simulink model "control_filtro_dq_mod2"  (R2017b)
settings: Solver=ode1  StartTime=0.0  StopTime=0.5  FixedStep=Ts  MaxStep=1e-4  RelTol=1e-3
InitFcn:
  | GlobalParam
values from neighbouring files (symbols this model uses):
  APFon = 0.025    [GlobalParam.m]
  Cdc = 680e-6    (= 0.00068)    [GlobalParam.m]
  fc = 15000    [GlobalParam.m]
  fe = 50    [GlobalParam.m]
  Ideal = 0    [GlobalParam.m]
  Lf = 0.01    [GlobalParam.m]
  LL = 0.055462    [GlobalParam.m]
  nc = 3    [GlobalParam.m]
  Rf = 0.35    [GlobalParam.m]
  RL = 23.232    [GlobalParam.m]
  teta_a = 0    [GlobalParam.m]
  teta_b = 120    [GlobalParam.m]
  teta_c = -120    [GlobalParam.m]
  Tm = 1/fm    (= 5e-05)    [GlobalParam.m]
  Ts = 5e-6    (= 5e-06)    [GlobalParam.m]
  Vdc = 62    [GlobalParam.m]
  Vs = 120*sqrt(2)    [GlobalParam.m]
libraries: powerlib x106, simulink x10, cstblocks x3, peTransforms x2, peSinusoidalMeasurement x1, powerlib_meascontrol x1
(part 1 of 2)
settings Model: Creator=user  LastModifiedBy=user

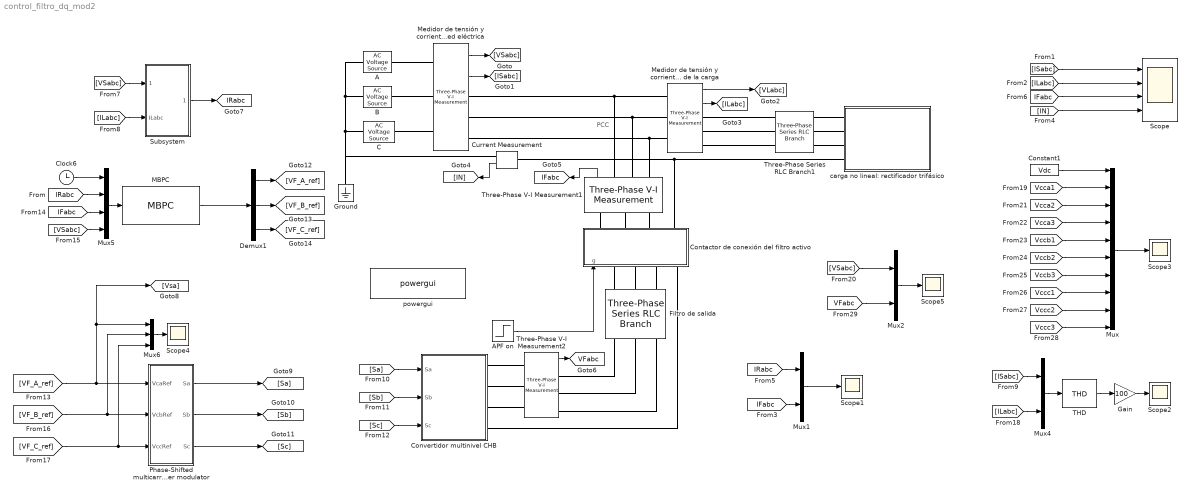
== system control_filtro_dq_mod2 ==
  note: PCC
  "A " : powerlib/Electrical Sources/AC Voltage Source  Amplitude=Vs  Phase=teta_a  Frequency=fe  SampleTime=0  Measurements=None  BusType=swing  Pref=10e3  Qref=0  Qmin=-inf  Qmax=+inf
  APF on : Step  Time=APFon  SampleTime=0
  "B " : powerlib/Electrical Sources/AC Voltage Source  Amplitude=Vs  Phase=teta_b  Frequency=fe  SampleTime=0  Measurements=None  BusType=swing  Pref=10e3  Qref=0  Qmin=-inf  Qmax=+inf
  "C " : powerlib/Electrical Sources/AC Voltage Source  Amplitude=Vs  Phase=teta_c  Frequency=fe  SampleTime=0  Measurements=None  BusType=swing  Pref=10e3  Qref=0  Qmin=-inf  Qmax=+inf
  Clock6 : Clock
  Constant1 : Constant  Value=Vdc
  "Contactor de conexión del filtro activo " : Subsystem
  Convertidor multinivel CHB : Subsystem
  Current Measurement : powerlib/Measurements/Current Measurement  PhasorSimulation=off  OutputType=Complex  PSBequivalent=0
  Demux1 : Demux  Outputs=3
  Filtro de salida : powerlib/Elements/Three-Phase Series RLC Branch  LConnTagsString=A|B|C  RConnTagsString=A|B|C  BranchType=RL  Resistance=Rf  Inductance=Lf  Capacitance=1e-6  Measurements=None
  Gain : Gain  Gain=100
  Ground : powerlib/Elements/Ground  LConnTagsString=a
  MBPC : MATLABFcn  MATLABFcn=MBPC  OutputDimensions=3
  Medidor de tensión y corriente de la red eléctrica : powerlib/Measurements/Three-Phase V-I Measurement  VoltageMeasurement=phase-to-ground  SetLabelV=off  LabelV=Vabc  Vpu=off  VpuLL=off  CurrentMeasurement=yes  SetLabelI=off  LabelI=Iabc  Ipu=off  Pbase=100e6  Vbase=500e3  OutputType=Complex  PhasorSimulation=off  PSBequivalent=0
  "Medidor de tensión y corriente de la carga " : powerlib/Measurements/Three-Phase V-I Measurement  VoltageMeasurement=phase-to-ground  SetLabelV=off  LabelV=Vabc  Vpu=off  VpuLL=off  CurrentMeasurement=yes  SetLabelI=off  LabelI=Iabc  Ipu=off  Pbase=100e6  Vbase=500e3  OutputType=Complex  PhasorSimulation=off  PSBequivalent=0
  Mux : Mux  Inputs=10
  Mux1 : Mux  Inputs=2
  Mux2 : Mux  Inputs=2
  Mux4 : Mux  Inputs=2
  Mux5 : Mux
  Mux6 : Mux  Inputs=3
  Phase-Shifted multicarrier modulator : Subsystem
  Scope : Scope  NumInputPorts=4
  Scope{1..5} (5 alike) : Scope
  Subsystem : Subsystem
  THD : powerlib_meascontrol/Measurements/THD  Freq=50  Ts=Ts
  Three-Phase Series RLC Branch1 : powerlib/Elements/Three-Phase Series RLC Branch  LConnTagsString=A|B|C  RConnTagsString=A|B|C  BranchType=RL  Resistance=0.09  Inductance=0.001  Capacitance=1e-6  Measurements=None
  Three-Phase V-I Measurement1 : powerlib/Measurements/Three-Phase V-I Measurement  VoltageMeasurement=no  SetLabelV=off  LabelV=Vabc  Vpu=off  VpuLL=off  CurrentMeasurement=yes  SetLabelI=off  LabelI=Iabc  Ipu=off  Pbase=100e6  Vbase=500e3  OutputType=Complex  PhasorSimulation=off  PSBequivalent=0
  Three-Phase V-I Measurement2 : powerlib/Measurements/Three-Phase V-I Measurement  VoltageMeasurement=phase-to-ground  SetLabelV=off  LabelV=Vabc  Vpu=off  VpuLL=off  CurrentMeasurement=no  SetLabelI=off  LabelI=Iabc  Ipu=off  Pbase=100e6  Vbase=500e3  OutputType=Complex  PhasorSimulation=off  PSBequivalent=0
  "carga no lineal: rectificador trifásico " : Subsystem
  powergui : powerlib/powergui  Priority=1  SimulationMode=Discrete  SampleTime=Ts  frequency=60  Iterations=50  frequencyindice=50  Pbase=100e6  ErrMax=1e-4  UnitsV=kV  UnitsW=MW  buscounter=0  FunctionMessages=off  echomessages=off  EnableUseOfTLC=off  CurrentSourceSwitches=off  DisableSnubberDevices=off  DisableRonSwitches=off  DisableVfSwitches=off  DisplayEquations=off  SolverType=Tustin/Backward Euler (TBE)  Interpol=off  ExternalGateDelay=off  methode=off  Ts=100  x0status=blocks  SPID=on  SwTol=0  HookPort=off  RestoreLinks=warning  ResistiveCurrentMeasurement=off  Frange=[0:2:500]  Ylog=off  Xlog=on  ShowGrid=off  save=off  variable=ZData  structure=vg11  ZoomFFT=off  StartTime=0.04  cycles=2  DisplayStyle=1  fundamental=50  FreqAxis=on  MaxFrequency=30000  frequencyindicesteady=1  RmsSteady=1  display=off
  tag scope: IFabc=global, IRabc=global, VFabc=global
  wires:
  Medidor de tensión y corriente de la red eléctrica/1 -> [VSabc]
  Medidor de tensión y corriente de la red eléctrica/2 -> [ISabc]
  "Medidor de tensión y corriente de la carga "/1 -> [VLabc]
  "Medidor de tensión y corriente de la carga "/2 -> [ILabc]
  [ILabc] -> Scope/2
  APF on/1 -> "Contactor de conexión del filtro activo "/1(g)
  Current Measurement/1 -> [IN]
  Three-Phase V-I Measurement1/1 -> [IFabc]
  Three-Phase V-I Measurement2/1 -> [VFabc]
  Mux5/1 -> MBPC/1
  MBPC/1 -> Demux1/1
  Clock6/1 -> Mux5/1
  [IRabc] -> Mux5/2
  [VSabc] -> Mux5/4
  [Sa] -> Convertidor multinivel CHB/1(Sa)
  [Sb] -> Convertidor multinivel CHB/2(Sb)
  [Sc] -> Convertidor multinivel CHB/3(Sc)
  [IFabc] -> Scope/3
  [IN] -> Scope/4
  [ISabc] -> Scope/1
  [IFabc] -> Mux5/3
  [IFabc] -> Mux1/2
  [IRabc] -> Mux1/1
  Mux1/1 -> Scope1/1
  [ISabc] -> Mux4/1
  Mux4/1 -> THD/1
  [ILabc] -> Mux4/2
  [Vccc1] -> Mux/8
  [Vcca1] -> Mux/2
  Constant1/1 -> Mux/1
  [Vccc2] -> Mux/9
  [Vccb2] -> Mux/6
  [Vccb1] -> Mux/5
  [Vccc3] -> Mux/10
  Mux/1 -> Scope3/1
  [Vccb3] -> Mux/7
  [Vcca3] -> Mux/4
  [Vcca2] -> Mux/3
  Demux1/1 -> [VF_A_ref]
  Demux1/2 -> [VF_B_ref]
  Demux1/3 -> [VF_C_ref]
  [VSabc] -> Mux2/1
  Mux2/1 -> Scope5/1
  THD/1 -> Gain/1
  Gain/1 -> Scope2/1
  [ILabc] -> Subsystem/2("ILabc ")
  [VSabc] -> Subsystem/1("VSabc ")
  Subsystem/1(IRabc1) -> [IRabc]
  [VFabc] -> Mux2/2
  Phase-Shifted multicarrier modulator/3(Sc) -> [Sc]
  Phase-Shifted multicarrier modulator/1(Sa) -> [Sa]
  Phase-Shifted multicarrier modulator/2(Sb) -> [Sb]
  Mux6/1 -> Scope4/1
  [VF_C_ref] -> Mux6/3, Phase-Shifted multicarrier modulator/3(VccRef)
  [VF_B_ref] -> Mux6/2, Phase-Shifted multicarrier modulator/2(VcbRef)
  [VF_A_ref] -> [Vsa], Mux6/1, Phase-Shifted multicarrier modulator/1(VcaRef)
  connections:
  "C "/LConn1 -- Ground/LConn1 -- Current Measurement/RConn1 -- "A "/LConn1 -- "B "/LConn1
  Medidor de tensión y corriente de la red eléctrica/LConn2 -- "B "/RConn1
  Medidor de tensión y corriente de la red eléctrica/LConn3 -- "C "/RConn1
  Medidor de tensión y corriente de la red eléctrica/LConn1 -- "A "/RConn1
  "Medidor de tensión y corriente de la carga "/LConn1 -- Three-Phase V-I Measurement1/RConn1 -- Medidor de tensión y corriente de la red eléctrica/RConn1
  "Medidor de tensión y corriente de la carga "/LConn2 -- Three-Phase V-I Measurement1/RConn2 -- Medidor de tensión y corriente de la red eléctrica/RConn2
  Medidor de tensión y corriente de la red eléctrica/RConn3 -- "Medidor de tensión y corriente de la carga "/LConn3 -- Three-Phase V-I Measurement1/RConn3
  Three-Phase Series RLC Branch1/LConn1 -- "Medidor de tensión y corriente de la carga "/RConn1
  Three-Phase Series RLC Branch1/LConn2 -- "Medidor de tensión y corriente de la carga "/RConn2
  Three-Phase Series RLC Branch1/LConn3 -- "Medidor de tensión y corriente de la carga "/RConn3
  Filtro de salida/RConn1 -- "Contactor de conexión del filtro activo "/LConn1
  "Contactor de conexión del filtro activo "/LConn2 -- Filtro de salida/RConn2
  Filtro de salida/RConn3 -- "Contactor de conexión del filtro activo "/LConn3
  Current Measurement/LConn1 -- "carga no lineal: rectificador trifásico "/LConn4 -- "Contactor de conexión del filtro activo "/RConn4
  Three-Phase V-I Measurement2/RConn1 -- Filtro de salida/LConn1
  Three-Phase V-I Measurement2/RConn2 -- Filtro de salida/LConn2
  Three-Phase V-I Measurement2/RConn3 -- Filtro de salida/LConn3
  Three-Phase V-I Measurement2/LConn1 -- Convertidor multinivel CHB/RConn1
  Three-Phase V-I Measurement2/LConn2 -- Convertidor multinivel CHB/RConn2
  Three-Phase V-I Measurement2/LConn3 -- Convertidor multinivel CHB/RConn3
  "Contactor de conexión del filtro activo "/LConn4 -- Convertidor multinivel CHB/RConn4
  "Contactor de conexión del filtro activo "/RConn3 -- Three-Phase V-I Measurement1/LConn3
  "Contactor de conexión del filtro activo "/RConn2 -- Three-Phase V-I Measurement1/LConn2
  "Contactor de conexión del filtro activo "/RConn1 -- Three-Phase V-I Measurement1/LConn1
  "carga no lineal: rectificador trifásico "/LConn1 -- Three-Phase Series RLC Branch1/RConn1
  "carga no lineal: rectificador trifásico "/LConn2 -- Three-Phase Series RLC Branch1/RConn2
  Three-Phase Series RLC Branch1/RConn3 -- "carga no lineal: rectificador trifásico "/LConn3

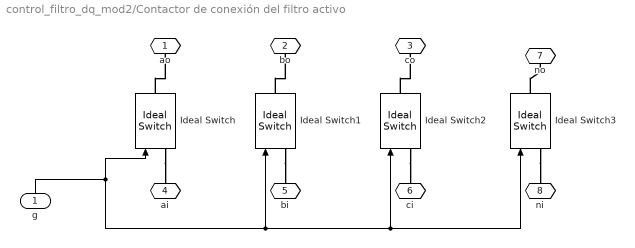
== system control_filtro_dq_mod2/Contactor de conexión del filtro activo  ==
  g : Inport
  Ideal Switch{,1..3} (4 alike) : powerlib/Power Electronics/Ideal Switch  Ron=0.001  Lon=0  IC=0  Rs=1e5  Cs=inf  Measurements=off
  ao : PMIOPort  Port=1  Side=Right
  bo : PMIOPort  Port=2  Side=Right
  co : PMIOPort  Port=3  Side=Right
  ai : PMIOPort  Port=4  Side=Left
  bi : PMIOPort  Port=5  Side=Left
  ci : PMIOPort  Port=6  Side=Left
  no : PMIOPort  Port=7  Side=Left
  ni : PMIOPort  Port=8  Side=Right
  wires:
  g/1 -> Ideal Switch3/1, Ideal Switch2/1, Ideal Switch1/1, Ideal Switch/1
  connections:
  Ideal Switch1/RConn1 -- bo/RConn1
  Ideal Switch1/LConn1 -- bi/RConn1
  Ideal Switch/RConn1 -- ao/RConn1
  Ideal Switch2/RConn1 -- co/RConn1
  Ideal Switch2/LConn1 -- ci/RConn1
  Ideal Switch/LConn1 -- ai/RConn1
  Ideal Switch3/LConn1 -- ni/RConn1
  Ideal Switch3/RConn1 -- no/RConn1

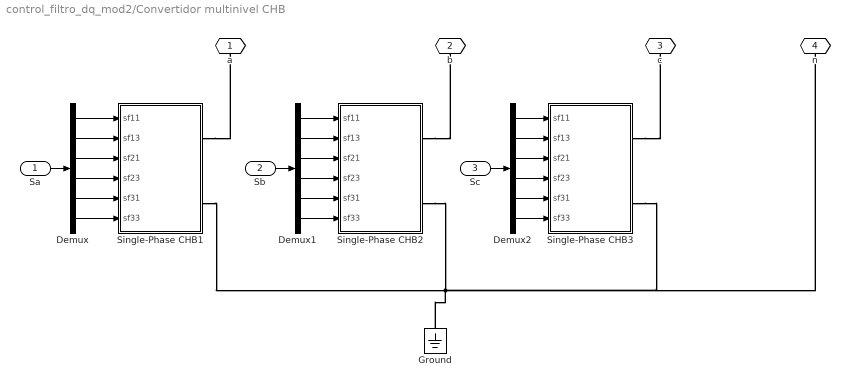
== system control_filtro_dq_mod2/Convertidor multinivel CHB ==
  Sa : Inport
  Sb : Inport  Port=2
  Sc : Inport  Port=3
  Demux : Demux  Outputs=6
  Demux1 : Demux  Outputs=6
  Demux2 : Demux  Outputs=6
  Ground : powerlib/Elements/Ground  LConnTagsString=a
  Single-Phase CHB1 : Subsystem
  Single-Phase CHB2 : Subsystem
  Single-Phase CHB3 : Subsystem
  a : PMIOPort  Port=1  Side=Right
  b : PMIOPort  Port=2  Side=Right
  c : PMIOPort  Port=3  Side=Right
  n : PMIOPort  Port=4  Side=Right
  wires:
  Demux/4 -> Single-Phase CHB1/4(sf23)
  Demux/6 -> Single-Phase CHB1/6(sf33)
  Demux/3 -> Single-Phase CHB1/3(sf21)
  Demux/2 -> Single-Phase CHB1/2(sf13)
  Demux/1 -> Single-Phase CHB1/1(sf11)
  Demux1/3 -> Single-Phase CHB2/3(sf21)
  Sa/1 -> Demux/1
  Sb/1 -> Demux1/1
  Sc/1 -> Demux2/1
  Demux2/1 -> Single-Phase CHB3/1(sf11)
  Demux1/1 -> Single-Phase CHB2/1(sf11)
  Demux1/6 -> Single-Phase CHB2/6(sf33)
  Demux2/6 -> Single-Phase CHB3/6(sf33)
  Demux/5 -> Single-Phase CHB1/5(sf31)
  Demux1/2 -> Single-Phase CHB2/2(sf13)
  Demux2/5 -> Single-Phase CHB3/5(sf31)
  Demux1/4 -> Single-Phase CHB2/4(sf23)
  Demux2/4 -> Single-Phase CHB3/4(sf23)
  Demux1/5 -> Single-Phase CHB2/5(sf31)
  Demux2/3 -> Single-Phase CHB3/3(sf21)
  Demux2/2 -> Single-Phase CHB3/2(sf13)
  connections:
  Single-Phase CHB2/RConn1 -- b/RConn1
  Single-Phase CHB1/RConn2 -- Ground/LConn1 -- Single-Phase CHB2/RConn2 -- Single-Phase CHB3/RConn2 -- n/RConn1
  Single-Phase CHB1/RConn1 -- a/RConn1
  Single-Phase CHB3/RConn1 -- c/RConn1

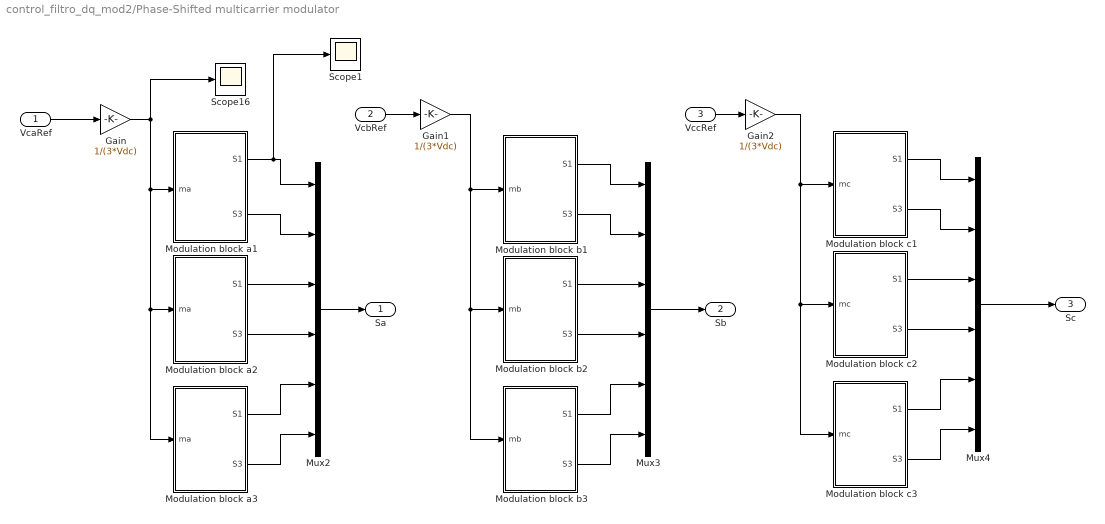
== system control_filtro_dq_mod2/Phase-Shifted multicarrier modulator ==
  VcaRef : Inport
  VcbRef : Inport  Port=2
  VccRef : Inport  Port=3
  Gain : Gain  Gain=1/(3*Vdc)
  Gain1 : Gain  Gain=1/(3*Vdc)
  Gain2 : Gain  Gain=1/(3*Vdc)
  Modulation block a1 : Subsystem
  Modulation block a2 : Subsystem
  Modulation block a3 : Subsystem
  Modulation block b1 : Subsystem
  Modulation block b2 : Subsystem
  Modulation block b3 : Subsystem
  Modulation block c1 : Subsystem
  Modulation block c2 : Subsystem
  Modulation block c3 : Subsystem
  Mux2 : Mux  Inputs=6
  Mux3 : Mux  Inputs=6
  Mux4 : Mux  Inputs=6
  Scope1 : Scope
  Scope16 : Scope
  Sa : Outport
  Sb : Outport  Port=2
  Sc : Outport  Port=3
  wires:
  Gain1/1 -> Modulation block b1/1(mb), Modulation block b2/1(mb), Modulation block b3/1(mb)
  Gain2/1 -> Modulation block c1/1(mc), Modulation block c2/1(mc), Modulation block c3/1(mc)
  Gain/1 -> Modulation block a1/1(ma), Modulation block a3/1(ma), Modulation block a2/1(ma), Scope16/1
  Modulation block a2/2(S3) -> Mux2/4
  Modulation block a2/1(S1) -> Mux2/3
  Modulation block a3/1(S1) -> Mux2/5
  Modulation block a3/2(S3) -> Mux2/6
  Modulation block a1/2(S3) -> Mux2/2
  Mux2/1 -> Sa/1
  Modulation block b2/2(S3) -> Mux3/4
  Modulation block b3/1(S1) -> Mux3/5
  Modulation block b3/2(S3) -> Mux3/6
  Modulation block b2/1(S1) -> Mux3/3
  Modulation block b1/2(S3) -> Mux3/2
  Modulation block b1/1(S1) -> Mux3/1
  Modulation block c3/1(S1) -> Mux4/5
  Modulation block c2/1(S1) -> Mux4/3
  Modulation block c2/2(S3) -> Mux4/4
  Mux4/1 -> Sc/1
  Modulation block c1/2(S3) -> Mux4/2
  Modulation block c1/1(S1) -> Mux4/1
  Modulation block c3/2(S3) -> Mux4/6
  Mux3/1 -> Sb/1
  VcbRef/1 -> Gain1/1
  VccRef/1 -> Gain2/1
  VcaRef/1 -> Gain/1
  Modulation block a1/1(S1) -> Scope1/1, Mux2/1

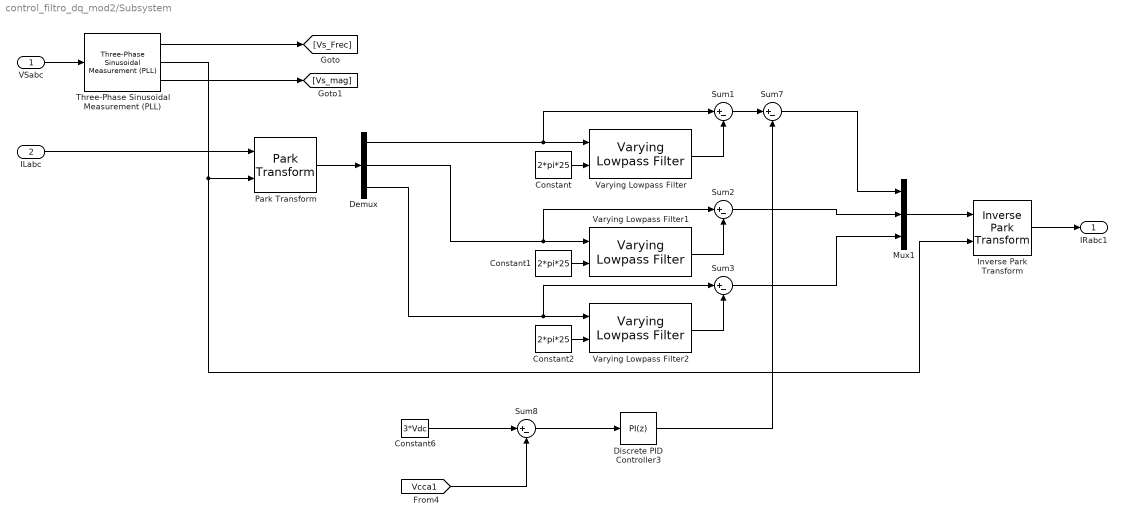
== system control_filtro_dq_mod2/Subsystem ==
  "VSabc " : Inport
  "ILabc " : Inport  Port=2
  Constant : Constant  Value=2*pi*25
  Constant1 : Constant  Value=2*pi*25
  Constant2 : Constant  Value=2*pi*25
  Constant6 : Constant  Value=3*Vdc
  Demux : Demux  Outputs=3
  Discrete PID Controller3 : simulink/Continuous/PID Controller  Controller=PI  TimeDomain=Discrete-time  SampleTime=1/5000  IntegratorMethod=Backward Euler  FilterMethod=Forward Euler  Form=Parallel  UseFilter=on  ControllerParametersSource=internal  P=0.0055  I=0.0009  D=0  N=100  InitialConditionSource=internal  InitialConditionForIntegrator=0  InitialConditionForFilter=0  ExternalReset=none  LimitOutput=off  UpperSaturationLimit=inf  LowerSaturationLimit=-inf  LinearizeAsGain=off  AntiWindupMode=none  Kb=1  TrackingMode=off  Kt=1  PParamMin=[]  PParamMax=[]  IParamMin=[]  IParamMax=[]  DParamMin=[]  DParamMax=[]  NParamMin=[]  NParamMax=[]  KbParamMin=[]  KbParamMax=[]  KtParamMin=[]  KtParamMax=[]  POutMin=[]  POutMax=[]  IOutMin=[]  IOutMax=[]  DOutMin=[]  DOutMax=[]  NOutMin=[]  NOutMax=[]  KbOutMin=[]  KbOutMax=[]  KtOutMin=[]  KtOutMax=[]  IntegratorOutMin=[]  IntegratorOutMax=[]  FilterOutMin=[]  FilterOutMax=[]  SumOutMin=[]  SumOutMax=[]  SumI1OutMin=[]  SumI1OutMax=[]  SumI2OutMin=[]  SumI2OutMax=[]  SumI3OutMin=[]  SumI3OutMax=[]  SumDOutMin=[]  SumDOutMax=[]  SaturationOutMin=[]  SaturationOutMax=[]  IntegratorContinuousStateAttributes=''  IntegratorStateMustResolveToSignalObject=off  IntegratorRTWStateStorageClass=Auto  FilterContinuousStateAttributes=''  FilterStateMustResolveToSignalObject=off  FilterRTWStateStorageClass=Auto  DifferentiatorICPrevScaledInput=0  DifferentiatorOutMin=[]  DifferentiatorOutMax=[]  InitialConditionSetting=State (most efficient)  FilterDiffOutCoefMin=[]  FilterDiffOutCoefMax=[]  SumDenOutMin=[]  SumDenOutMax=[]  SumNumOutMin=[]  SumNumOutMax=[]  ReciprocalOutMin=[]  ReciprocalOutMax=[]  DivideOutMin=[]  DivideOutMax=[]  TunerSelectOption=Transfer Function Based (PID Tuner App)
  Inverse Park Transform : peTransforms/Inverse Park Transform  AxisAlignment=D-axis  PowerInvariant=on
  Mux1 : Mux  Inputs=3
  Park Transform : peTransforms/Park Transform  AxisAlignment=D-axis  PowerInvariant=on
  Sum{1..3,7..8} (5 alike) : Sum  Inputs=|+-
  Three-Phase Sinusoidal Measurement (PLL) : peSinusoidalMeasurement/Three-Phase Sinusoidal Measurement (PLL)  Kp_LF=200  Ki_LF=2000  F0=50  Theta0=0  Ts=Ts
  Varying Lowpass Filter : cstblocks/Linear Parameter Varying/Varying Lowpass Filter  N=2
      settings: SourceProductName=Control System Toolbox
  Varying Lowpass Filter1 : cstblocks/Linear Parameter Varying/Varying Lowpass Filter  N=2
      settings: SourceProductName=Control System Toolbox
  Varying Lowpass Filter2 : cstblocks/Linear Parameter Varying/Varying Lowpass Filter  N=2
      settings: SourceProductName=Control System Toolbox
  IRabc1 : Outport
  wires:
  Constant/1 -> Varying Lowpass Filter/2
  Inverse Park Transform/1 -> IRabc1/1
  "VSabc "/1 -> Three-Phase Sinusoidal Measurement (PLL)/1
  Three-Phase Sinusoidal Measurement (PLL)/2 -> Park Transform/2, Inverse Park Transform/2
  "ILabc "/1 -> Park Transform/1
  Three-Phase Sinusoidal Measurement (PLL)/1 -> [Vs_Frec]
  Park Transform/1 -> Demux/1
  Mux1/1 -> Inverse Park Transform/1
  Three-Phase Sinusoidal Measurement (PLL)/3 -> [Vs_mag]
  Demux/1 -> Sum1/1, Varying Lowpass Filter/1
  Varying Lowpass Filter/1 -> Sum1/2
  Sum1/1 -> Sum7/1
  Sum7/1 -> Mux1/1
  Sum8/1 -> Discrete PID Controller3/1
  Constant6/1 -> Sum8/1
  Discrete PID Controller3/1 -> Sum7/2
  Constant1/1 -> Varying Lowpass Filter1/2
  Demux/2 -> Sum2/1, Varying Lowpass Filter1/1
  Varying Lowpass Filter1/1 -> Sum2/2
  Sum2/1 -> Mux1/2
  Constant2/1 -> Varying Lowpass Filter2/2
  Varying Lowpass Filter2/1 -> Sum3/2
  Demux/3 -> Sum3/1, Varying Lowpass Filter2/1
  Sum3/1 -> Mux1/3
  [Vcca1] -> Sum8/2

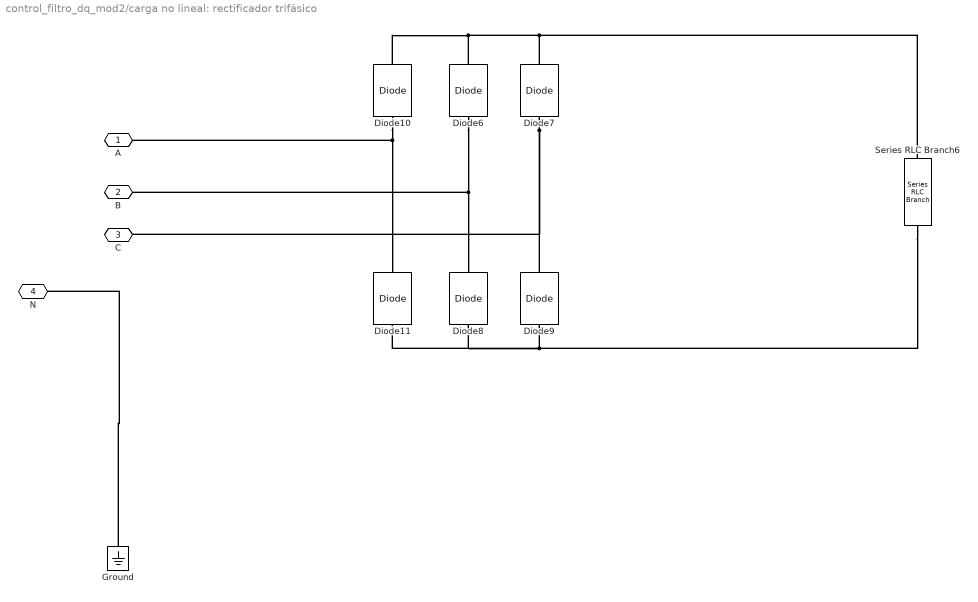
== system control_filtro_dq_mod2/carga no lineal: rectificador trifásico  ==
  Diode{6..11} (6 alike) : powerlib/Power Electronics/Diode  Ron=0.001  Lon=0  Vf=0  IC=0  UseSnubber=off  Rs=500  Cs=250e-9  Measurements=off
  Ground : powerlib/Elements/Ground  LConnTagsString=a
  Series RLC Branch6 : powerlib/Elements/Series RLC Branch  LConnTagsString=__new0  RConnTagsString=__new0  BranchType=RL  Resistance=RL*4  Inductance=LL*2  SetiL0=off  InitialCurrent=0  Capacitance=1e-6  Setx0=off  InitialVoltage=0  Measurements=None
  "A " : PMIOPort  Port=1  Side=Left
  B : PMIOPort  Port=2  Side=Left
  "C " : PMIOPort  Port=3  Side=Left
  "N " : PMIOPort  Port=4  Side=Left
  connections:
  Ground/LConn1 -- "N "/RConn1
  Diode7/RConn1 -- Series RLC Branch6/LConn1 -- Diode10/RConn1 -- Diode6/RConn1
  Diode10/LConn1 -- Diode11/RConn1 -- "A "/RConn1
  Series RLC Branch6/RConn1 -- Diode9/LConn1 -- Diode8/LConn1 -- Diode11/LConn1
  Diode6/LConn1 -- B/RConn1 -- Diode8/RConn1
  Diode7/LConn1 -- "C "/RConn1 -- Diode9/RConn1

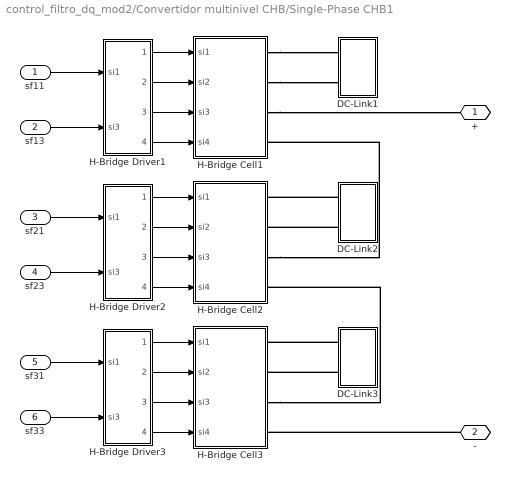
== system control_filtro_dq_mod2/Convertidor multinivel CHB/Single-Phase CHB1 ==
  sf11 : Inport
  sf13 : Inport  Port=2
  sf21 : Inport  Port=3
  sf23 : Inport  Port=4
  sf31 : Inport  Port=5
  sf33 : Inport  Port=6
  DC-Link1 : Subsystem
  DC-Link2 : Subsystem
  DC-Link3 : Subsystem
  H-Bridge Cell1 : Subsystem
  H-Bridge Cell2 : Subsystem
  H-Bridge Cell3 : Subsystem
  H-Bridge Driver1 : Subsystem
  H-Bridge Driver2 : Subsystem
  H-Bridge Driver3 : Subsystem
  + : PMIOPort  Port=1  Side=Right
  - : PMIOPort  Port=2  Side=Right
  wires:
  H-Bridge Driver2/1(1) -> H-Bridge Cell2/1(si1)
  H-Bridge Driver2/3(3) -> H-Bridge Cell2/3(si3)
  H-Bridge Driver2/2(2) -> H-Bridge Cell2/2(si2)
  H-Bridge Driver2/4(4) -> H-Bridge Cell2/4(si4)
  H-Bridge Driver1/1(1) -> H-Bridge Cell1/1(si1)
  H-Bridge Driver1/2(2) -> H-Bridge Cell1/2(si2)
  H-Bridge Driver1/3(3) -> H-Bridge Cell1/3(si3)
  H-Bridge Driver1/4(4) -> H-Bridge Cell1/4(si4)
  sf23/1 -> H-Bridge Driver2/2(si3)
  sf13/1 -> H-Bridge Driver1/2(si3)
  sf21/1 -> H-Bridge Driver2/1(si1)
  sf31/1 -> H-Bridge Driver3/1(si1)
  sf11/1 -> H-Bridge Driver1/1(si1)
  sf33/1 -> H-Bridge Driver3/2(si3)
  H-Bridge Driver3/2(2) -> H-Bridge Cell3/2(si2)
  H-Bridge Driver3/1(1) -> H-Bridge Cell3/1(si1)
  H-Bridge Driver3/3(3) -> H-Bridge Cell3/3(si3)
  H-Bridge Driver3/4(4) -> H-Bridge Cell3/4(si4)
  connections:
  H-Bridge Cell2/RConn3 -- H-Bridge Cell1/RConn4
  DC-Link2/RConn2 -- H-Bridge Cell2/RConn2
  DC-Link2/RConn1 -- H-Bridge Cell2/RConn1
  H-Bridge Cell1/RConn1 -- DC-Link1/RConn1
  H-Bridge Cell1/RConn2 -- DC-Link1/RConn2
  H-Bridge Cell1/RConn3 -- +/RConn1
  -/RConn1 -- H-Bridge Cell3/RConn4
  H-Bridge Cell3/RConn3 -- H-Bridge Cell2/RConn4
  DC-Link3/RConn2 -- H-Bridge Cell3/RConn2
  DC-Link3/RConn1 -- H-Bridge Cell3/RConn1

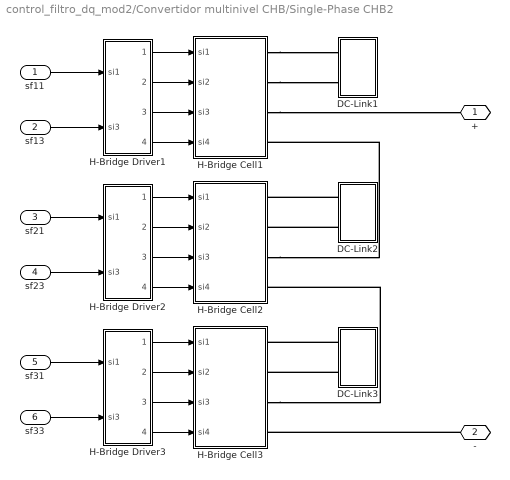
== system control_filtro_dq_mod2/Convertidor multinivel CHB/Single-Phase CHB2 ==
  sf11 : Inport
  sf13 : Inport  Port=2
  sf21 : Inport  Port=3
  sf23 : Inport  Port=4
  sf31 : Inport  Port=5
  sf33 : Inport  Port=6
  DC-Link1 : Subsystem
  DC-Link2 : Subsystem
  DC-Link3 : Subsystem
  H-Bridge Cell1 : Subsystem
  H-Bridge Cell2 : Subsystem
  H-Bridge Cell3 : Subsystem
  H-Bridge Driver1 : Subsystem
  H-Bridge Driver2 : Subsystem
  H-Bridge Driver3 : Subsystem
  + : PMIOPort  Port=1  Side=Right
  - : PMIOPort  Port=2  Side=Right
  wires:
  H-Bridge Driver2/1(1) -> H-Bridge Cell2/1(si1)
  H-Bridge Driver2/3(3) -> H-Bridge Cell2/3(si3)
  H-Bridge Driver2/2(2) -> H-Bridge Cell2/2(si2)
  H-Bridge Driver2/4(4) -> H-Bridge Cell2/4(si4)
  H-Bridge Driver1/1(1) -> H-Bridge Cell1/1(si1)
  H-Bridge Driver1/2(2) -> H-Bridge Cell1/2(si2)
  H-Bridge Driver1/3(3) -> H-Bridge Cell1/3(si3)
  H-Bridge Driver1/4(4) -> H-Bridge Cell1/4(si4)
  sf23/1 -> H-Bridge Driver2/2(si3)
  sf13/1 -> H-Bridge Driver1/2(si3)
  sf21/1 -> H-Bridge Driver2/1(si1)
  sf31/1 -> H-Bridge Driver3/1(si1)
  sf11/1 -> H-Bridge Driver1/1(si1)
  sf33/1 -> H-Bridge Driver3/2(si3)
  H-Bridge Driver3/2(2) -> H-Bridge Cell3/2(si2)
  H-Bridge Driver3/1(1) -> H-Bridge Cell3/1(si1)
  H-Bridge Driver3/3(3) -> H-Bridge Cell3/3(si3)
  H-Bridge Driver3/4(4) -> H-Bridge Cell3/4(si4)
  connections:
  H-Bridge Cell2/RConn3 -- H-Bridge Cell1/RConn4
  DC-Link2/RConn2 -- H-Bridge Cell2/RConn2
  DC-Link2/RConn1 -- H-Bridge Cell2/RConn1
  H-Bridge Cell1/RConn1 -- DC-Link1/RConn1
  H-Bridge Cell1/RConn2 -- DC-Link1/RConn2
  H-Bridge Cell1/RConn3 -- +/RConn1
  -/RConn1 -- H-Bridge Cell3/RConn4
  H-Bridge Cell3/RConn3 -- H-Bridge Cell2/RConn4
  DC-Link3/RConn2 -- H-Bridge Cell3/RConn2
  DC-Link3/RConn1 -- H-Bridge Cell3/RConn1

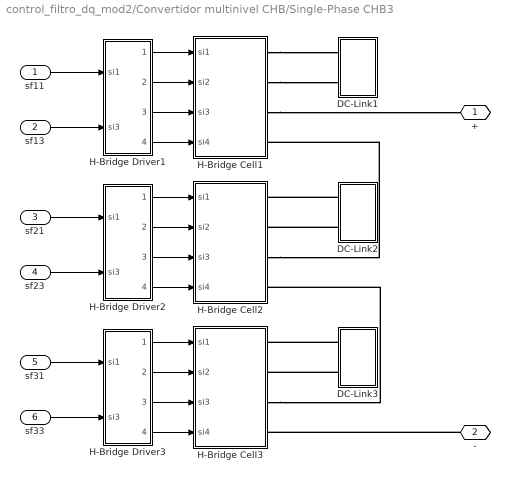
== system control_filtro_dq_mod2/Convertidor multinivel CHB/Single-Phase CHB3 ==
  sf11 : Inport
  sf13 : Inport  Port=2
  sf21 : Inport  Port=3
  sf23 : Inport  Port=4
  sf31 : Inport  Port=5
  sf33 : Inport  Port=6
  DC-Link1 : Subsystem
  DC-Link2 : Subsystem
  DC-Link3 : Subsystem
  H-Bridge Cell1 : Subsystem
  H-Bridge Cell2 : Subsystem
  H-Bridge Cell3 : Subsystem
  H-Bridge Driver1 : Subsystem
  H-Bridge Driver2 : Subsystem
  H-Bridge Driver3 : Subsystem
  + : PMIOPort  Port=1  Side=Right
  - : PMIOPort  Port=2  Side=Right
  wires:
  H-Bridge Driver2/1(1) -> H-Bridge Cell2/1(si1)
  H-Bridge Driver2/3(3) -> H-Bridge Cell2/3(si3)
  H-Bridge Driver2/2(2) -> H-Bridge Cell2/2(si2)
  H-Bridge Driver2/4(4) -> H-Bridge Cell2/4(si4)
  H-Bridge Driver1/1(1) -> H-Bridge Cell1/1(si1)
  H-Bridge Driver1/2(2) -> H-Bridge Cell1/2(si2)
  H-Bridge Driver1/3(3) -> H-Bridge Cell1/3(si3)
  H-Bridge Driver1/4(4) -> H-Bridge Cell1/4(si4)
  sf23/1 -> H-Bridge Driver2/2(si3)
  sf13/1 -> H-Bridge Driver1/2(si3)
  sf21/1 -> H-Bridge Driver2/1(si1)
  sf31/1 -> H-Bridge Driver3/1(si1)
  sf11/1 -> H-Bridge Driver1/1(si1)
  sf33/1 -> H-Bridge Driver3/2(si3)
  H-Bridge Driver3/2(2) -> H-Bridge Cell3/2(si2)
  H-Bridge Driver3/1(1) -> H-Bridge Cell3/1(si1)
  H-Bridge Driver3/3(3) -> H-Bridge Cell3/3(si3)
  H-Bridge Driver3/4(4) -> H-Bridge Cell3/4(si4)
  connections:
  H-Bridge Cell2/RConn3 -- H-Bridge Cell1/RConn4
  DC-Link2/RConn2 -- H-Bridge Cell2/RConn2
  DC-Link2/RConn1 -- H-Bridge Cell2/RConn1
  H-Bridge Cell1/RConn1 -- DC-Link1/RConn1
  H-Bridge Cell1/RConn2 -- DC-Link1/RConn2
  H-Bridge Cell1/RConn3 -- +/RConn1
  -/RConn1 -- H-Bridge Cell3/RConn4
  H-Bridge Cell3/RConn3 -- H-Bridge Cell2/RConn4
  DC-Link3/RConn2 -- H-Bridge Cell3/RConn2
  DC-Link3/RConn1 -- H-Bridge Cell3/RConn1

== system control_filtro_dq_mod2/Phase-Shifted multicarrier modulator/Modulation block a1 ==
  ma : Inport
  Data Type Conversion : DataTypeConversion  OutDataTypeStr=double
  Data Type Conversion3 : DataTypeConversion  OutDataTypeStr=double
  Gain1 : Gain  Gain=-1
  Relational Operator : RelationalOperator  Operator=<=  OutDataTypeStr=boolean  RndMeth=Nearest
  Relational Operator2 : RelationalOperator  Operator=<=  OutDataTypeStr=boolean  RndMeth=Nearest
  Repeating Sequence1 : simulink/Sources/Repeating Sequence  rep_seq_t="[0 (1/fc)/2  1/fc]"  rep_seq_y=[-1 1 -1]
  Scope : Scope
  S1 : Outport
  S3 : Outport  Port=2
  wires:
  Relational Operator/1 -> Data Type Conversion/1
  Repeating Sequence1/1 -> Scope/1, Relational Operator/1, Relational Operator2/1
  Data Type Conversion/1 -> S1/1
  ma/1 -> Relational Operator/2, Gain1/1
  Relational Operator2/1 -> Data Type Conversion3/1
  Data Type Conversion3/1 -> S3/1
  Gain1/1 -> Relational Operator2/2

== system control_filtro_dq_mod2/Phase-Shifted multicarrier modulator/Modulation block a2 ==
  ma : Inport
  Data Type Conversion : DataTypeConversion  OutDataTypeStr=double
  Data Type Conversion3 : DataTypeConversion  OutDataTypeStr=double
  Gain1 : Gain  Gain=-1
  Relational Operator : RelationalOperator  Operator=<=  OutDataTypeStr=boolean  RndMeth=Nearest
  Relational Operator2 : RelationalOperator  Operator=<=  OutDataTypeStr=boolean  RndMeth=Nearest
  Repeating Sequence1 : simulink/Sources/Repeating Sequence  rep_seq_t="[0 (1/fc)/2  1/fc]"  rep_seq_y=[-1 1 -1]
  Transport Delay : TransportDelay  DelayTime=Tm*(180/nc)/360
  S1 : Outport
  S3 : Outport  Port=2
  wires:
  Relational Operator/1 -> Data Type Conversion/1
  Repeating Sequence1/1 -> Transport Delay/1
  Data Type Conversion/1 -> S1/1
  ma/1 -> Relational Operator/2, Gain1/1
  Relational Operator2/1 -> Data Type Conversion3/1
  Data Type Conversion3/1 -> S3/1
  Gain1/1 -> Relational Operator2/2
  Transport Delay/1 -> Relational Operator/1, Relational Operator2/1

== system control_filtro_dq_mod2/Phase-Shifted multicarrier modulator/Modulation block a3 ==
  ma : Inport
  Data Type Conversion : DataTypeConversion  OutDataTypeStr=double
  Data Type Conversion3 : DataTypeConversion  OutDataTypeStr=double
  Gain1 : Gain  Gain=-1
  Relational Operator : RelationalOperator  Operator=<=  OutDataTypeStr=boolean  RndMeth=Nearest
  Relational Operator2 : RelationalOperator  Operator=<=  OutDataTypeStr=boolean  RndMeth=Nearest
  Repeating Sequence1 : simulink/Sources/Repeating Sequence  rep_seq_t="[0 (1/fc)/2  1/fc]"  rep_seq_y=[-1 1 -1]
  Transport Delay : TransportDelay  DelayTime=(Tm*(180/nc)/360)*2
  S1 : Outport
  S3 : Outport  Port=2
  wires:
  Relational Operator/1 -> Data Type Conversion/1
  Repeating Sequence1/1 -> Transport Delay/1
  Data Type Conversion/1 -> S1/1
  ma/1 -> Relational Operator/2, Gain1/1
  Relational Operator2/1 -> Data Type Conversion3/1
  Data Type Conversion3/1 -> S3/1
  Gain1/1 -> Relational Operator2/2
  Transport Delay/1 -> Relational Operator/1, Relational Operator2/1

== system control_filtro_dq_mod2/Phase-Shifted multicarrier modulator/Modulation block b1 ==
  mb : Inport
  Data Type Conversion : DataTypeConversion  OutDataTypeStr=double
  Data Type Conversion3 : DataTypeConversion  OutDataTypeStr=double
  Gain1 : Gain  Gain=-1
  Relational Operator : RelationalOperator  Operator=<=  OutDataTypeStr=boolean  RndMeth=Nearest
  Relational Operator2 : RelationalOperator  Operator=<=  OutDataTypeStr=boolean  RndMeth=Nearest
  Repeating Sequence1 : simulink/Sources/Repeating Sequence  rep_seq_t="[0 (1/fc)/2  1/fc]"  rep_seq_y=[-1 1 -1]
  S1 : Outport
  S3 : Outport  Port=2
  wires:
  Relational Operator/1 -> Data Type Conversion/1
  Repeating Sequence1/1 -> Relational Operator/1, Relational Operator2/1
  Data Type Conversion/1 -> S1/1
  mb/1 -> Relational Operator/2, Gain1/1
  Relational Operator2/1 -> Data Type Conversion3/1
  Data Type Conversion3/1 -> S3/1
  Gain1/1 -> Relational Operator2/2

== system control_filtro_dq_mod2/Phase-Shifted multicarrier modulator/Modulation block b2 ==
  mb : Inport
  Data Type Conversion : DataTypeConversion  OutDataTypeStr=double
  Data Type Conversion3 : DataTypeConversion  OutDataTypeStr=double
  Gain1 : Gain  Gain=-1
  Relational Operator : RelationalOperator  Operator=<=  OutDataTypeStr=boolean  RndMeth=Nearest
  Relational Operator2 : RelationalOperator  Operator=<=  OutDataTypeStr=boolean  RndMeth=Nearest
  Repeating Sequence1 : simulink/Sources/Repeating Sequence  rep_seq_t="[0 (1/fc)/2  1/fc]"  rep_seq_y=[-1 1 -1]
  Transport Delay : TransportDelay  DelayTime=Tm*(180/nc)/360
  S1 : Outport
  S3 : Outport  Port=2
  wires:
  Relational Operator/1 -> Data Type Conversion/1
  Repeating Sequence1/1 -> Transport Delay/1
  Data Type Conversion/1 -> S1/1
  mb/1 -> Relational Operator/2, Gain1/1
  Relational Operator2/1 -> Data Type Conversion3/1
  Data Type Conversion3/1 -> S3/1
  Gain1/1 -> Relational Operator2/2
  Transport Delay/1 -> Relational Operator/1, Relational Operator2/1

== system control_filtro_dq_mod2/Phase-Shifted multicarrier modulator/Modulation block b3 ==
  mb : Inport
  Data Type Conversion : DataTypeConversion  OutDataTypeStr=double
  Data Type Conversion3 : DataTypeConversion  OutDataTypeStr=double
  Gain1 : Gain  Gain=-1
  Relational Operator : RelationalOperator  Operator=<=  OutDataTypeStr=boolean  RndMeth=Nearest
  Relational Operator2 : RelationalOperator  Operator=<=  OutDataTypeStr=boolean  RndMeth=Nearest
  Repeating Sequence1 : simulink/Sources/Repeating Sequence  rep_seq_t="[0 (1/fc)/2  1/fc]"  rep_seq_y=[-1 1 -1]
  Transport Delay : TransportDelay  DelayTime=(Tm*(180/nc)/360)*2
  S1 : Outport
  S3 : Outport  Port=2
  wires:
  Relational Operator/1 -> Data Type Conversion/1
  Repeating Sequence1/1 -> Transport Delay/1
  Data Type Conversion/1 -> S1/1
  mb/1 -> Relational Operator/2, Gain1/1
  Relational Operator2/1 -> Data Type Conversion3/1
  Data Type Conversion3/1 -> S3/1
  Gain1/1 -> Relational Operator2/2
  Transport Delay/1 -> Relational Operator/1, Relational Operator2/1

== system control_filtro_dq_mod2/Phase-Shifted multicarrier modulator/Modulation block c1 ==
  mc : Inport
  Data Type Conversion : DataTypeConversion  OutDataTypeStr=double
  Data Type Conversion3 : DataTypeConversion  OutDataTypeStr=double
  Gain1 : Gain  Gain=-1
  Relational Operator : RelationalOperator  Operator=<=  OutDataTypeStr=boolean  RndMeth=Nearest
  Relational Operator2 : RelationalOperator  Operator=<=  OutDataTypeStr=boolean  RndMeth=Nearest
  Repeating Sequence1 : simulink/Sources/Repeating Sequence  rep_seq_t="[0 (1/fc)/2  1/fc]"  rep_seq_y=[-1 1 -1]
  S1 : Outport
  S3 : Outport  Port=2
  wires:
  Relational Operator/1 -> Data Type Conversion/1
  Repeating Sequence1/1 -> Relational Operator/1, Relational Operator2/1
  Data Type Conversion/1 -> S1/1
  mc/1 -> Relational Operator/2, Gain1/1
  Relational Operator2/1 -> Data Type Conversion3/1
  Data Type Conversion3/1 -> S3/1
  Gain1/1 -> Relational Operator2/2

== system control_filtro_dq_mod2/Phase-Shifted multicarrier modulator/Modulation block c2 ==
  mc : Inport
  Data Type Conversion : DataTypeConversion  OutDataTypeStr=double
  Data Type Conversion3 : DataTypeConversion  OutDataTypeStr=double
  Gain1 : Gain  Gain=-1
  Relational Operator : RelationalOperator  Operator=<=  OutDataTypeStr=boolean  RndMeth=Nearest
  Relational Operator2 : RelationalOperator  Operator=<=  OutDataTypeStr=boolean  RndMeth=Nearest
  Repeating Sequence1 : simulink/Sources/Repeating Sequence  rep_seq_t="[0 (1/fc)/2  1/fc]"  rep_seq_y=[-1 1 -1]
  Transport Delay : TransportDelay  DelayTime=(Tm*(180/nc)/360)*2
  S1 : Outport
  S3 : Outport  Port=2
  wires:
  Relational Operator/1 -> Data Type Conversion/1
  Repeating Sequence1/1 -> Transport Delay/1
  Data Type Conversion/1 -> S1/1
  mc/1 -> Relational Operator/2, Gain1/1
  Relational Operator2/1 -> Data Type Conversion3/1
  Data Type Conversion3/1 -> S3/1
  Gain1/1 -> Relational Operator2/2
  Transport Delay/1 -> Relational Operator/1, Relational Operator2/1

== system control_filtro_dq_mod2/Phase-Shifted multicarrier modulator/Modulation block c3 ==
  mc : Inport
  Data Type Conversion : DataTypeConversion  OutDataTypeStr=double
  Data Type Conversion3 : DataTypeConversion  OutDataTypeStr=double
  Gain1 : Gain  Gain=-1
  Relational Operator : RelationalOperator  Operator=<=  OutDataTypeStr=boolean  RndMeth=Nearest
  Relational Operator2 : RelationalOperator  Operator=<=  OutDataTypeStr=boolean  RndMeth=Nearest
  Repeating Sequence1 : simulink/Sources/Repeating Sequence  rep_seq_t="[0 (1/fc)/2  1/fc]"  rep_seq_y=[-1 1 -1]
  Transport Delay : TransportDelay  DelayTime=(Tm*(180/nc)/360)*2
  S1 : Outport
  S3 : Outport  Port=2
  wires:
  Relational Operator/1 -> Data Type Conversion/1
  Repeating Sequence1/1 -> Transport Delay/1
  Data Type Conversion/1 -> S1/1
  mc/1 -> Relational Operator/2, Gain1/1
  Relational Operator2/1 -> Data Type Conversion3/1
  Data Type Conversion3/1 -> S3/1
  Gain1/1 -> Relational Operator2/2
  Transport Delay/1 -> Relational Operator/1, Relational Operator2/1

== system control_filtro_dq_mod2/Convertidor multinivel CHB/Single-Phase CHB1/DC-Link1 ==
  Constant : Constant  Value=Ideal
  DC Capacitor : powerlib/Elements/Series RLC Branch  LConnTagsString=__new0  RConnTagsString=__new0  BranchType=C  Resistance=0.09  Inductance=0.002996  SetiL0=off  InitialCurrent=0  Capacitance=Cdc  Setx0=on  InitialVoltage=Vodc  Measurements=None
  DC Voltage Source : powerlib/Electrical Sources/DC Voltage Source  Amplitude=Vdc  Measurements=None
  Ideal Switch : powerlib/Power Electronics/Ideal Switch  Ron=0.001  Lon=0  IC=0  Rs=1e5  Cs=inf  Measurements=off
  Ideal Switch2 : powerlib/Power Electronics/Ideal Switch  Ron=0.001  Lon=0  IC=0  Rs=1e5  Cs=inf  Measurements=off
  Logical Operator2 : Logic  Operator=NOT  AllPortsSameDT=off  OutDataTypeStr=boolean
  Vcan3 : powerlib/Measurements/Voltage Measurement  PhasorSimulation=off  OutputType=Complex  PSBequivalent=0
  + : PMIOPort  Port=1  Side=Right
  - : PMIOPort  Port=2  Side=Right
  tag scope: Vcca1=global
  wires:
  Constant/1 -> Ideal Switch/1, Logical Operator2/1
  Logical Operator2/1 -> Ideal Switch2/1
  Vcan3/1 -> [Vcca1]
  connections:
  Ideal Switch/RConn1 -- Ideal Switch2/RConn1 -- Vcan3/LConn1 -- +/RConn1
  DC Voltage Source/RConn1 -- Ideal Switch/LConn1
  -/RConn1 -- Vcan3/LConn2 -- DC Voltage Source/LConn1 -- DC Capacitor/RConn1
  Ideal Switch2/LConn1 -- DC Capacitor/LConn1

== system control_filtro_dq_mod2/Convertidor multinivel CHB/Single-Phase CHB1/DC-Link2 ==
  Constant : Constant  Value=Ideal
  DC Capacitor : powerlib/Elements/Series RLC Branch  LConnTagsString=__new0  RConnTagsString=__new0  BranchType=C  Resistance=0.09  Inductance=0.002996  SetiL0=off  InitialCurrent=0  Capacitance=Cdc  Setx0=on  InitialVoltage=Vodc  Measurements=None
  DC Voltage Source : powerlib/Electrical Sources/DC Voltage Source  Amplitude=Vdc  Measurements=None
  Ideal Switch : powerlib/Power Electronics/Ideal Switch  Ron=0.001  Lon=0  IC=0  Rs=1e5  Cs=inf  Measurements=off
  Ideal Switch2 : powerlib/Power Electronics/Ideal Switch  Ron=0.001  Lon=0  IC=0  Rs=1e5  Cs=inf  Measurements=off
  Logical Operator2 : Logic  Operator=NOT  AllPortsSameDT=off  OutDataTypeStr=boolean
  Vcan3 : powerlib/Measurements/Voltage Measurement  PhasorSimulation=off  OutputType=Complex  PSBequivalent=0
  + : PMIOPort  Port=1  Side=Right
  - : PMIOPort  Port=2  Side=Right
  tag scope: Vcca2=global
  wires:
  Constant/1 -> Ideal Switch/1, Logical Operator2/1
  Logical Operator2/1 -> Ideal Switch2/1
  Vcan3/1 -> [Vcca2]
  connections:
  Ideal Switch/RConn1 -- Ideal Switch2/RConn1 -- Vcan3/LConn1 -- +/RConn1
  DC Voltage Source/RConn1 -- Ideal Switch/LConn1
  -/RConn1 -- DC Capacitor/RConn1 -- DC Voltage Source/LConn1 -- Vcan3/LConn2
  Ideal Switch2/LConn1 -- DC Capacitor/LConn1

== system control_filtro_dq_mod2/Convertidor multinivel CHB/Single-Phase CHB1/DC-Link3 ==
  Constant : Constant  Value=Ideal
  DC Capacitor : powerlib/Elements/Series RLC Branch  LConnTagsString=__new0  RConnTagsString=__new0  BranchType=C  Resistance=0.09  Inductance=0.002996  SetiL0=off  InitialCurrent=0  Capacitance=Cdc  Setx0=on  InitialVoltage=Vodc  Measurements=None
  DC Voltage Source : powerlib/Electrical Sources/DC Voltage Source  Amplitude=Vdc  Measurements=None
  Ideal Switch : powerlib/Power Electronics/Ideal Switch  Ron=0.001  Lon=0  IC=0  Rs=1e5  Cs=inf  Measurements=off
  Ideal Switch2 : powerlib/Power Electronics/Ideal Switch  Ron=0.001  Lon=0  IC=0  Rs=1e5  Cs=inf  Measurements=off
  Logical Operator2 : Logic  Operator=NOT  AllPortsSameDT=off  OutDataTypeStr=boolean
  Vcan3 : powerlib/Measurements/Voltage Measurement  PhasorSimulation=off  OutputType=Complex  PSBequivalent=0
  + : PMIOPort  Port=1  Side=Right
  - : PMIOPort  Port=2  Side=Right
  tag scope: Vcca3=global
  wires:
  Constant/1 -> Ideal Switch/1, Logical Operator2/1
  Logical Operator2/1 -> Ideal Switch2/1
  Vcan3/1 -> [Vcca3]
  connections:
  Ideal Switch/RConn1 -- Ideal Switch2/RConn1 -- Vcan3/LConn1 -- +/RConn1
  DC Voltage Source/RConn1 -- Ideal Switch/LConn1
  -/RConn1 -- Vcan3/LConn2 -- DC Capacitor/RConn1 -- DC Voltage Source/LConn1
  DC Capacitor/LConn1 -- Ideal Switch2/LConn1

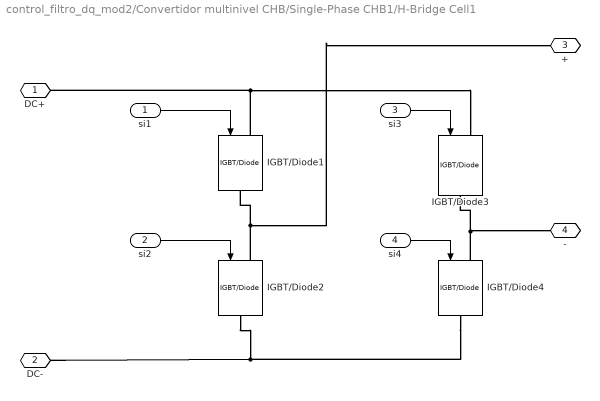
== system control_filtro_dq_mod2/Convertidor multinivel CHB/Single-Phase CHB1/H-Bridge Cell1 ==
  si1 : Inport
  si2 : Inport  Port=2
  si3 : Inport  Port=3
  si4 : Inport  Port=4
  IGBT/Diode{1..4} (4 alike) : powerlib/Power Electronics/IGBT//Diode  Ron=Ron  Rs=Rs  Cs=Cs  Measurements=off
  DC+ : PMIOPort  Port=1  Side=Right
  DC- : PMIOPort  Port=2  Side=Right
  + : PMIOPort  Port=3  Side=Right
  - : PMIOPort  Port=4  Side=Right
  wires:
  si4/1 -> IGBT/Diode4/1
  si2/1 -> IGBT/Diode2/1
  si3/1 -> IGBT/Diode3/1
  si1/1 -> IGBT/Diode1/1
  connections:
  IGBT/Diode3/RConn1 -- IGBT/Diode4/LConn1 -- -/RConn1
  DC-/RConn1 -- IGBT/Diode4/RConn1 -- IGBT/Diode2/RConn1
  IGBT/Diode1/RConn1 -- IGBT/Diode2/LConn1 -- +/RConn1
  IGBT/Diode1/LConn1 -- IGBT/Diode3/LConn1 -- DC+/RConn1

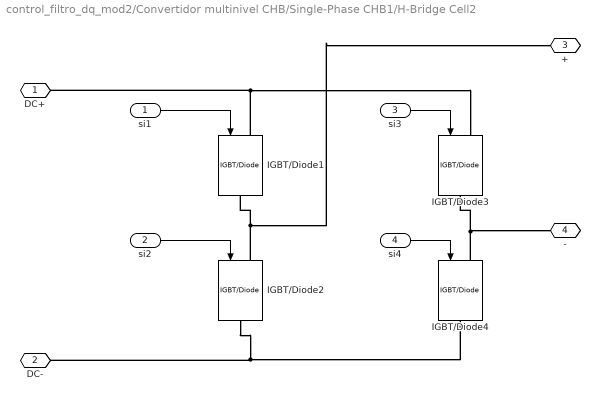
== system control_filtro_dq_mod2/Convertidor multinivel CHB/Single-Phase CHB1/H-Bridge Cell2 ==
  si1 : Inport
  si2 : Inport  Port=2
  si3 : Inport  Port=3
  si4 : Inport  Port=4
  IGBT/Diode{1..4} (4 alike) : powerlib/Power Electronics/IGBT//Diode  Ron=Ron  Rs=Rs  Cs=Cs  Measurements=off
  DC+ : PMIOPort  Port=1  Side=Right
  DC- : PMIOPort  Port=2  Side=Right
  + : PMIOPort  Port=3  Side=Right
  - : PMIOPort  Port=4  Side=Right
  wires:
  si4/1 -> IGBT/Diode4/1
  si2/1 -> IGBT/Diode2/1
  si3/1 -> IGBT/Diode3/1
  si1/1 -> IGBT/Diode1/1
  connections:
  IGBT/Diode3/RConn1 -- IGBT/Diode4/LConn1 -- -/RConn1
  IGBT/Diode2/RConn1 -- IGBT/Diode4/RConn1 -- DC-/RConn1
  IGBT/Diode1/RConn1 -- IGBT/Diode2/LConn1 -- +/RConn1
  IGBT/Diode1/LConn1 -- IGBT/Diode3/LConn1 -- DC+/RConn1

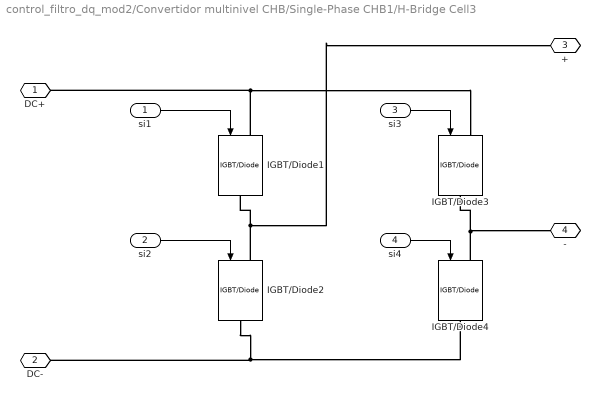
== system control_filtro_dq_mod2/Convertidor multinivel CHB/Single-Phase CHB1/H-Bridge Cell3 ==
  si1 : Inport
  si2 : Inport  Port=2
  si3 : Inport  Port=3
  si4 : Inport  Port=4
  IGBT/Diode{1..4} (4 alike) : powerlib/Power Electronics/IGBT//Diode  Ron=Ron  Rs=Rs  Cs=Cs  Measurements=off
  DC+ : PMIOPort  Port=1  Side=Right
  DC- : PMIOPort  Port=2  Side=Right
  + : PMIOPort  Port=3  Side=Right
  - : PMIOPort  Port=4  Side=Right
  wires:
  si4/1 -> IGBT/Diode4/1
  si2/1 -> IGBT/Diode2/1
  si3/1 -> IGBT/Diode3/1
  si1/1 -> IGBT/Diode1/1
  connections:
  IGBT/Diode3/RConn1 -- IGBT/Diode4/LConn1 -- -/RConn1
  IGBT/Diode2/RConn1 -- IGBT/Diode4/RConn1 -- DC-/RConn1
  IGBT/Diode1/RConn1 -- IGBT/Diode2/LConn1 -- +/RConn1
  IGBT/Diode1/LConn1 -- IGBT/Diode3/LConn1 -- DC+/RConn1

== system control_filtro_dq_mod2/Convertidor multinivel CHB/Single-Phase CHB1/H-Bridge Driver1 ==
  si1 : Inport
  si3 : Inport  Port=2
  Logical Operator2 : Logic  Operator=NOT  AllPortsSameDT=off  OutDataTypeStr=boolean
  Logical Operator3 : Logic  Operator=NOT  AllPortsSameDT=off  OutDataTypeStr=boolean
  1 : Outport
  2 : Outport  Port=2
  3 : Outport  Port=3
  4 : Outport  Port=4
  wires:
  si3/1 -> 3/1, Logical Operator3/1
  si1/1 -> 1/1, Logical Operator2/1
  Logical Operator3/1 -> 4/1
  Logical Operator2/1 -> 2/1

== system control_filtro_dq_mod2/Convertidor multinivel CHB/Single-Phase CHB1/H-Bridge Driver2 ==
  si1 : Inport
  si3 : Inport  Port=2
  Logical Operator2 : Logic  Operator=NOT  AllPortsSameDT=off  OutDataTypeStr=boolean
  Logical Operator3 : Logic  Operator=NOT  AllPortsSameDT=off  OutDataTypeStr=boolean
  1 : Outport
  2 : Outport  Port=2
  3 : Outport  Port=3
  4 : Outport  Port=4
  wires:
  si3/1 -> 3/1, Logical Operator3/1
  si1/1 -> 1/1, Logical Operator2/1
  Logical Operator3/1 -> 4/1
  Logical Operator2/1 -> 2/1

== system control_filtro_dq_mod2/Convertidor multinivel CHB/Single-Phase CHB1/H-Bridge Driver3 ==
  si1 : Inport
  si3 : Inport  Port=2
  Logical Operator2 : Logic  Operator=NOT  AllPortsSameDT=off  OutDataTypeStr=boolean
  Logical Operator3 : Logic  Operator=NOT  AllPortsSameDT=off  OutDataTypeStr=boolean
  1 : Outport
  2 : Outport  Port=2
  3 : Outport  Port=3
  4 : Outport  Port=4
  wires:
  si3/1 -> 3/1, Logical Operator3/1
  si1/1 -> 1/1, Logical Operator2/1
  Logical Operator3/1 -> 4/1
  Logical Operator2/1 -> 2/1

== system control_filtro_dq_mod2/Convertidor multinivel CHB/Single-Phase CHB2/DC-Link1 ==
  Constant : Constant  Value=Ideal
  DC Capacitor : powerlib/Elements/Series RLC Branch  LConnTagsString=__new0  RConnTagsString=__new0  BranchType=C  Resistance=0.09  Inductance=0.002996  SetiL0=off  InitialCurrent=0  Capacitance=Cdc  Setx0=on  InitialVoltage=Vodc  Measurements=None
  DC Voltage Source : powerlib/Electrical Sources/DC Voltage Source  Amplitude=Vdc  Measurements=None
  Ideal Switch : powerlib/Power Electronics/Ideal Switch  Ron=0.001  Lon=0  IC=0  Rs=1e5  Cs=inf  Measurements=off
  Ideal Switch2 : powerlib/Power Electronics/Ideal Switch  Ron=0.001  Lon=0  IC=0  Rs=1e5  Cs=inf  Measurements=off
  Logical Operator2 : Logic  Operator=NOT  AllPortsSameDT=off  OutDataTypeStr=boolean
  Vcan3 : powerlib/Measurements/Voltage Measurement  PhasorSimulation=off  OutputType=Complex  PSBequivalent=0
  + : PMIOPort  Port=1  Side=Right
  - : PMIOPort  Port=2  Side=Right
  tag scope: Vccb1=global
  wires:
  Constant/1 -> Ideal Switch/1, Logical Operator2/1
  Logical Operator2/1 -> Ideal Switch2/1
  Vcan3/1 -> [Vccb1]
  connections:
  Ideal Switch/RConn1 -- Ideal Switch2/RConn1 -- Vcan3/LConn1 -- +/RConn1
  DC Voltage Source/RConn1 -- Ideal Switch/LConn1
  -/RConn1 -- Vcan3/LConn2 -- DC Voltage Source/LConn1 -- DC Capacitor/RConn1
  Ideal Switch2/LConn1 -- DC Capacitor/LConn1

== system control_filtro_dq_mod2/Convertidor multinivel CHB/Single-Phase CHB2/DC-Link2 ==
  Constant : Constant  Value=Ideal
  DC Capacitor : powerlib/Elements/Series RLC Branch  LConnTagsString=__new0  RConnTagsString=__new0  BranchType=C  Resistance=0.09  Inductance=0.002996  SetiL0=off  InitialCurrent=0  Capacitance=Cdc  Setx0=on  InitialVoltage=Vodc  Measurements=None
  DC Voltage Source : powerlib/Electrical Sources/DC Voltage Source  Amplitude=Vdc  Measurements=None
  Ideal Switch : powerlib/Power Electronics/Ideal Switch  Ron=0.001  Lon=0  IC=0  Rs=1e5  Cs=inf  Measurements=off
  Ideal Switch2 : powerlib/Power Electronics/Ideal Switch  Ron=0.001  Lon=0  IC=0  Rs=1e5  Cs=inf  Measurements=off
  Logical Operator2 : Logic  Operator=NOT  AllPortsSameDT=off  OutDataTypeStr=boolean
  Vcan3 : powerlib/Measurements/Voltage Measurement  PhasorSimulation=off  OutputType=Complex  PSBequivalent=0
  + : PMIOPort  Port=1  Side=Right
  - : PMIOPort  Port=2  Side=Right
  tag scope: Vccb2=global
  wires:
  Constant/1 -> Ideal Switch/1, Logical Operator2/1
  Vcan3/1 -> [Vccb2]
  Logical Operator2/1 -> Ideal Switch2/1
  connections:
  Ideal Switch/RConn1 -- Ideal Switch2/RConn1 -- Vcan3/LConn1 -- +/RConn1
  DC Voltage Source/RConn1 -- Ideal Switch/LConn1
  -/RConn1 -- DC Capacitor/RConn1 -- DC Voltage Source/LConn1 -- Vcan3/LConn2
  Ideal Switch2/LConn1 -- DC Capacitor/LConn1

== system control_filtro_dq_mod2/Convertidor multinivel CHB/Single-Phase CHB2/DC-Link3 ==
  Constant : Constant  Value=Ideal
  DC Capacitor : powerlib/Elements/Series RLC Branch  LConnTagsString=__new0  RConnTagsString=__new0  BranchType=C  Resistance=0.09  Inductance=0.002996  SetiL0=off  InitialCurrent=0  Capacitance=Cdc  Setx0=on  InitialVoltage=Vodc  Measurements=None
  DC Voltage Source : powerlib/Electrical Sources/DC Voltage Source  Amplitude=Vdc  Measurements=None
  Ideal Switch : powerlib/Power Electronics/Ideal Switch  Ron=0.001  Lon=0  IC=0  Rs=1e5  Cs=inf  Measurements=off
  Ideal Switch2 : powerlib/Power Electronics/Ideal Switch  Ron=0.001  Lon=0  IC=0  Rs=1e5  Cs=inf  Measurements=off
  Logical Operator2 : Logic  Operator=NOT  AllPortsSameDT=off  OutDataTypeStr=boolean
  Vcan3 : powerlib/Measurements/Voltage Measurement  PhasorSimulation=off  OutputType=Complex  PSBequivalent=0
  + : PMIOPort  Port=1  Side=Right
  - : PMIOPort  Port=2  Side=Right
  tag scope: Vccb3=global
  wires:
  Constant/1 -> Ideal Switch/1, Logical Operator2/1
  Logical Operator2/1 -> Ideal Switch2/1
  Vcan3/1 -> [Vccb3]
  connections:
  Ideal Switch/RConn1 -- Ideal Switch2/RConn1 -- Vcan3/LConn1 -- +/RConn1
  DC Voltage Source/RConn1 -- Ideal Switch/LConn1
  -/RConn1 -- Vcan3/LConn2 -- DC Capacitor/RConn1 -- DC Voltage Source/LConn1
  Ideal Switch2/LConn1 -- DC Capacitor/LConn1

== system control_filtro_dq_mod2/Convertidor multinivel CHB/Single-Phase CHB2/H-Bridge Cell1 ==
  si1 : Inport
  si2 : Inport  Port=2
  si3 : Inport  Port=3
  si4 : Inport  Port=4
  IGBT/Diode{1..4} (4 alike) : powerlib/Power Electronics/IGBT//Diode  Ron=Ron  Rs=Rs  Cs=Cs  Measurements=off
  DC+ : PMIOPort  Port=1  Side=Right
  DC- : PMIOPort  Port=2  Side=Right
  + : PMIOPort  Port=3  Side=Right
  - : PMIOPort  Port=4  Side=Right
  wires:
  si4/1 -> IGBT/Diode4/1
  si2/1 -> IGBT/Diode2/1
  si3/1 -> IGBT/Diode3/1
  si1/1 -> IGBT/Diode1/1
  connections:
  IGBT/Diode3/RConn1 -- -/RConn1 -- IGBT/Diode4/LConn1
  IGBT/Diode2/RConn1 -- DC-/RConn1 -- IGBT/Diode4/RConn1
  IGBT/Diode1/RConn1 -- +/RConn1 -- IGBT/Diode2/LConn1
  IGBT/Diode1/LConn1 -- IGBT/Diode3/LConn1 -- DC+/RConn1

== system control_filtro_dq_mod2/Convertidor multinivel CHB/Single-Phase CHB2/H-Bridge Cell2 ==
  si1 : Inport
  si2 : Inport  Port=2
  si3 : Inport  Port=3
  si4 : Inport  Port=4
  IGBT/Diode{1..4} (4 alike) : powerlib/Power Electronics/IGBT//Diode  Ron=Ron  Rs=Rs  Cs=Cs  Measurements=off
  DC+ : PMIOPort  Port=1  Side=Right
  DC- : PMIOPort  Port=2  Side=Right
  + : PMIOPort  Port=3  Side=Right
  - : PMIOPort  Port=4  Side=Right
  wires:
  si4/1 -> IGBT/Diode4/1
  si2/1 -> IGBT/Diode2/1
  si3/1 -> IGBT/Diode3/1
  si1/1 -> IGBT/Diode1/1
  connections:
  IGBT/Diode3/RConn1 -- IGBT/Diode4/LConn1 -- -/RConn1
  IGBT/Diode2/RConn1 -- IGBT/Diode4/RConn1 -- DC-/RConn1
  IGBT/Diode1/RConn1 -- IGBT/Diode2/LConn1 -- +/RConn1
  IGBT/Diode1/LConn1 -- IGBT/Diode3/LConn1 -- DC+/RConn1

== system control_filtro_dq_mod2/Convertidor multinivel CHB/Single-Phase CHB2/H-Bridge Cell3 ==
  si1 : Inport
  si2 : Inport  Port=2
  si3 : Inport  Port=3
  si4 : Inport  Port=4
  IGBT/Diode{1..4} (4 alike) : powerlib/Power Electronics/IGBT//Diode  Ron=Ron  Rs=Rs  Cs=Cs  Measurements=off
  DC+ : PMIOPort  Port=1  Side=Right
  DC- : PMIOPort  Port=2  Side=Right
  + : PMIOPort  Port=3  Side=Right
  - : PMIOPort  Port=4  Side=Right
  wires:
  si4/1 -> IGBT/Diode4/1
  si2/1 -> IGBT/Diode2/1
  si3/1 -> IGBT/Diode3/1
  si1/1 -> IGBT/Diode1/1
  connections:
  IGBT/Diode3/RConn1 -- IGBT/Diode4/LConn1 -- -/RConn1
  IGBT/Diode2/RConn1 -- IGBT/Diode4/RConn1 -- DC-/RConn1
  IGBT/Diode1/RConn1 -- IGBT/Diode2/LConn1 -- +/RConn1
  IGBT/Diode1/LConn1 -- IGBT/Diode3/LConn1 -- DC+/RConn1

== system control_filtro_dq_mod2/Convertidor multinivel CHB/Single-Phase CHB2/H-Bridge Driver1 ==
  si1 : Inport
  si3 : Inport  Port=2
  Logical Operator2 : Logic  Operator=NOT  AllPortsSameDT=off  OutDataTypeStr=boolean
  Logical Operator3 : Logic  Operator=NOT  AllPortsSameDT=off  OutDataTypeStr=boolean
  1 : Outport
  2 : Outport  Port=2
  3 : Outport  Port=3
  4 : Outport  Port=4
  wires:
  si3/1 -> 3/1, Logical Operator3/1
  si1/1 -> 1/1, Logical Operator2/1
  Logical Operator3/1 -> 4/1
  Logical Operator2/1 -> 2/1

== system control_filtro_dq_mod2/Convertidor multinivel CHB/Single-Phase CHB2/H-Bridge Driver2 ==
  si1 : Inport
  si3 : Inport  Port=2
  Logical Operator2 : Logic  Operator=NOT  AllPortsSameDT=off  OutDataTypeStr=boolean
  Logical Operator3 : Logic  Operator=NOT  AllPortsSameDT=off  OutDataTypeStr=boolean
  1 : Outport
  2 : Outport  Port=2
  3 : Outport  Port=3
  4 : Outport  Port=4
  wires:
  si3/1 -> 3/1, Logical Operator3/1
  si1/1 -> 1/1, Logical Operator2/1
  Logical Operator3/1 -> 4/1
  Logical Operator2/1 -> 2/1

== system control_filtro_dq_mod2/Convertidor multinivel CHB/Single-Phase CHB2/H-Bridge Driver3 ==
  si1 : Inport
  si3 : Inport  Port=2
  Logical Operator2 : Logic  Operator=NOT  AllPortsSameDT=off  OutDataTypeStr=boolean
  Logical Operator3 : Logic  Operator=NOT  AllPortsSameDT=off  OutDataTypeStr=boolean
  1 : Outport
  2 : Outport  Port=2
  3 : Outport  Port=3
  4 : Outport  Port=4
  wires:
  si3/1 -> 3/1, Logical Operator3/1
  si1/1 -> 1/1, Logical Operator2/1
  Logical Operator3/1 -> 4/1
  Logical Operator2/1 -> 2/1
